simulink model "tests"  (R2020b)
settings: Solver=VariableStepAuto  StartTime=0.0  StopTime=1  RelTol=1e-3
settings Model: Creator=kika  LastModifiedBy=kika

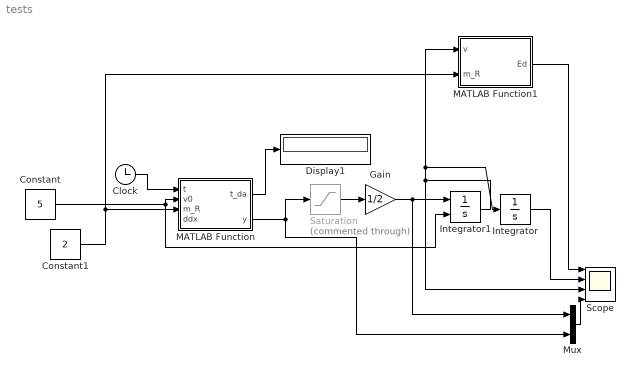
== system tests ==
  Clock : Clock
  Constant : Constant  Value=5
  Constant1 : Constant  Value=2
  Display1 : Display
  Gain : Gain  Gain=1/2
  Integrator : Integrator
  Integrator1 : Integrator  InitialConditionSource=external  InitialCondition=1
  MATLAB Function : MATLAB Function  TreatAsAtomicUnit=on
  MATLAB Function1 : MATLAB Function  TreatAsAtomicUnit=on
  Mux : Mux  Inputs=2
  Saturation : Saturate  Commented=through  UpperLimit=1  LowerLimit=-1
  Scope : Scope  NumInputPorts=4
  wires:
  Integrator1/1 -> MATLAB Function1/1(v), Integrator/1, Scope/3
  Clock/1 -> MATLAB Function/1(t)
  Constant/1 -> Integrator1/2, MATLAB Function/2(v0)
  Constant1/1 -> MATLAB Function1/2(m_R), MATLAB Function/3(m_R)
  MATLAB Function1/1(Ed) -> Scope/1
  MATLAB Function/1(t_da) -> Display1/1
  Gain/1 -> Mux/1, Integrator1/1
  Integrator/1 -> Scope/2
  Mux/1 -> Scope/4
  MATLAB Function/2(y) -> Mux/2, Saturation/1
  Saturation/1 -> Gain/1

== matlab function tests/MATLAB Function1 ==
  data: v input; Ed output; m_R input
function Ed = fcn(v, m_R)

    Ed = 0.5 * m_R * v;

== matlab function tests/MATLAB Function ==
  data: t_da output; t input; y output; v0 input; m_R input; ddx input
function [t_da, y]= fcn(t, v0, m_R, ddx)


    F_max = 6;
    a = F_max / m_R;
    
    t_da = v0 / a;
    
    y = 0;
    if t < t_da
        y = m_R * -a;
%         y = -m_R * ddx;
    end
    
%     
%     
%     
%     
%     v0 = 1;
%     x0 = 2;
%     x = 0;
% 
%     tda = (-v0 + sqrt(v0^2 + 2 * a * (x - x0))) / a;
%     
%     x = x0 - v0 * t + 0.5 * a * t^2;
%     v = v0 + a*t;
%     y=0;
%     
%     
%     xf = 1;
%     xs = 0;
    
%     tf = 3;
%     
%     v = 1.5 * (xf - xs) / tf;
%  
%     tb = (xs - xf + v*tf) / v;
%     a = -v / tb;
    
%     
%     v = v0;
%     a = a_max;
%     tf = v / a_max;
%     d = v * tf;
%     xf = d - xs;
%     tb = (xs - xf + v*tf) / v;
%     
%     
%     
%     if t <= tb
%         y = a * t;
%     elseif t > tb && t <= (tf - tb)
%         y = v;
%     elseif t > (tf - tb) && t <= tf
%         y = a* tf - a * t;
%     else
%         y = 0;
%     end
